simulink model "Predictor_de_smith"  (R2014a)
settings: Solver=ode45  StartTime=0.0  StopTime=1000  RelTol=1e-3
values from neighbouring files (symbols this model uses):
  Fh0 = 0.8946    [Seccion_4.m]    (also in backup_workspace.mat)
  Kc_Normal = 9.6108    [Seccion_4.m]    (also in backup_workspace.mat)
  Kc_Smith = 24.0269    [Seccion_4.m]    (also in backup_workspace.mat)
  Tau_Normal = 100    [Seccion_4.m]    (also in backup_workspace.mat)
  Tau_Smith = 100    [Seccion_4.m]    (also in backup_workspace.mat)
libraries: simulink_need_slupdate x2
settings Model: Creator=sebar  LastModifiedBy=sebar

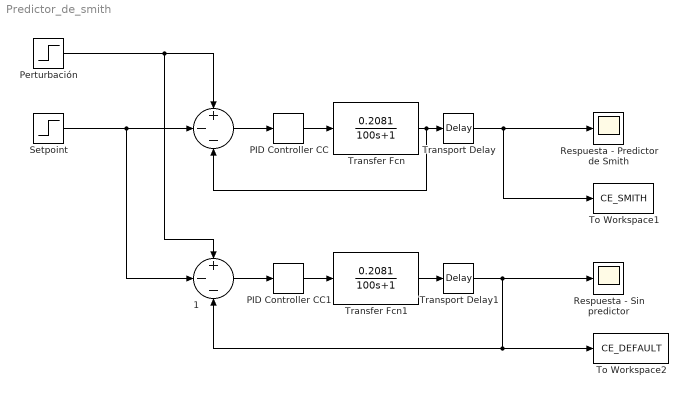
== system Predictor_de_smith ==
  " " : Sum  Inputs=+--
  " 1" : Sum  Inputs=+--
  PID Controller CC : simulink_need_slupdate/PID Controller  P=Kc_Smith  I=Kc_Smith/Tau_Smith  D=0
  PID Controller CC1 : simulink_need_slupdate/PID Controller  P=Kc_Normal  I=Kc_Normal/Tau_Normal  D=0
  Perturbación : Step  Time=100  Before=Fh0  After=Fh0*1.02  SampleTime=1
  "Respuesta - Predictor de Smith " : Scope
  Respuesta - Sin predictor : Scope
  Setpoint : Step  Time=0  Before=Fh0  After=Fh0  SampleTime=1
  To Workspace1 : ToWorkspace  VariableName=CE_SMITH  SaveFormat=Structure With Time
  To Workspace2 : ToWorkspace  VariableName=CE_DEFAULT  SaveFormat=Structure With Time
  Transfer Fcn : TransferFcn  Numerator=[0.2081]  Denominator=[100 1]
  Transfer Fcn1 : TransferFcn  Numerator=[0.2081]  Denominator=[100 1]
  Transport Delay : TransportDelay  DelayTime=21.8
  Transport Delay1 : TransportDelay  DelayTime=21.8
  wires:
  " "/1 -> PID Controller CC/1
  Transfer Fcn/1 -> " "/3, Transport Delay/1
  Transport Delay/1 -> "Respuesta - Predictor de Smith "/1, To Workspace1/1
  Setpoint/1 -> " 1"/2, " "/2
  PID Controller CC/1 -> Transfer Fcn/1
  Perturbación/1 -> " "/1, " 1"/1
  " 1"/1 -> PID Controller CC1/1
  Transfer Fcn1/1 -> Transport Delay1/1
  Transport Delay1/1 -> " 1"/3, To Workspace2/1, Respuesta - Sin predictor/1
  PID Controller CC1/1 -> Transfer Fcn1/1
